simulink model "overcurrentest"  (R2019b)
settings: Solver=ode45  StartTime=0.0  StopTime=1.0  RelTol=1e-3  AbsTol=1e-6
undefined symbols (not defined in the file or in its folder): Time
libraries: elements x36
settings Model: ExtModeTrigMode=oneshot  ExtModeArmWhenConnect=off  Creator=PC  LastModifiedBy=taif205
settings SolverCC: AutoScaleAbsTol=off
settings DataIOCC: SaveFormat=Array  SignalLoggingSaveFormat=ModelDataLogs  ReturnWorkspaceOutputs=off
settings OptimizationCC: BlockReduction=off  BooleanDataType=off  LifeSpan=inf
settings DebuggingCC: SaveWithParameterizedLinksMsg=none  UnderspecifiedInitializationDetection=Classic  MergeDetectMultiDrivingBlocksExec=none  SignalResolutionControl=TryResolveAllWithWarning  MultiTaskDSMMsg=warning  MultiTaskCondExecSysMsg=none  SFUnexpectedBacktrackingDiag=warning  SFNoUnconditionalDefaultTransitionDiag=warning  SFExecutionAtInitializationDiag=none  ArithmeticOperatorsInVariantConditions=warning
settings HardwareCC: ProdBitPerPointer=32  ProdBitPerSizeT=32  ProdBitPerPtrDiffT=32  ProdLargestAtomicFloat=None  ProdIntDivRoundTo=Undefined  ProdEndianess=Unspecified  ProdWordSize=32  ProdHWDeviceType=32-bit Generic  TargetUnknown=on
settings ModelReferenceCC: PropagateSignalLabelsOutOfModel=off
settings SFSimCC: SimUseLocalCustomCode=off  CustomCodeUndefinedFunction=UseInterfaceOnly
settings RTWCC: RTWUseLocalCustomCode=off
settings CodeAppCC: StateflowObjectComments=on
settings GRTTargetCC: TargetLangStandard=C89/C90 (ANSI)  GeneratePreprocessorConditionals=Disable all  CombineOutputUpdateFcns=off  GRTInterface=on
settings ConfigComp: CovMetricSettings=dw  CovHtmlReporting=on  CovSaveCumulativeToWorkspaceVar=on  CovSaveSingleToWorkspaceVar=on  CovExternalEMLEnable=off

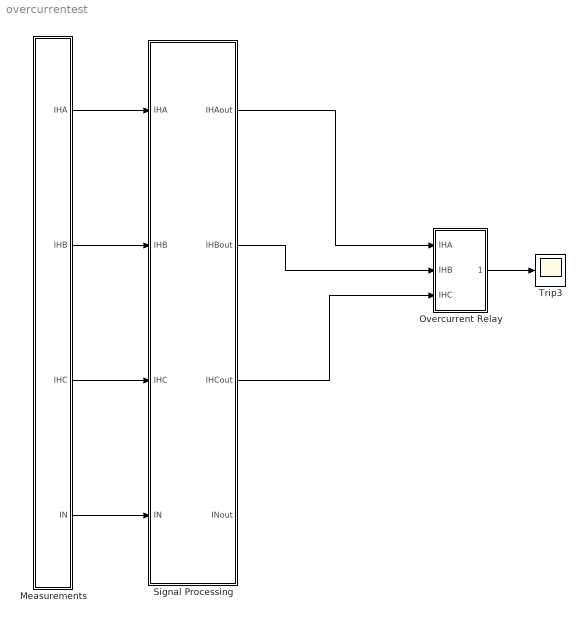
== system overcurrentest ==
  Measurements : Subsystem
  Overcurrent Relay : Subsystem  mask(Three-phase Inverse-time Overcurrent Relay){k=0.02, reset=0.9, pickupv=3}
      mask prompts: k "Time Parameter"; reset "Ratio of Reset to pick up"; pickupv "Pick-up Value"
      mask help: Three-phase inverse-time overcurrent relays for the back-up protection of the high voltage winding.
  Signal Processing : Subsystem  mask(Signal Processing){ctx=31.5, cth=1.38, vs=13.8e3, vp=315e3, vector=11}
      mask prompts: ctx "CT Ratio of Low Voltage Side"; cth "CT Ratio of High Voltage Side"; vs "Secondary Voltage"; vp "Primary Voltage"; vector "Transformer Connection Vector"
      mask help: Transform analog measurements to digital format, including filtering, sampling . . .
  Trip3 : Scope
  wires:
  Measurements/1(IHA) -> Signal Processing/1(IHA)
  Measurements/2(IHB) -> Signal Processing/2(IHB)
  Measurements/3(IHC) -> Signal Processing/3(IHC)
  Measurements/4(IN) -> Signal Processing/4(IN)
  Overcurrent Relay/1(Trip 3) -> Trip3/1
  Signal Processing/1(IHAout) -> Overcurrent Relay/1(IHA)
  Signal Processing/2(IHBout) -> Overcurrent Relay/2(IHB)
  Signal Processing/3(IHCout) -> Overcurrent Relay/3(IHC)

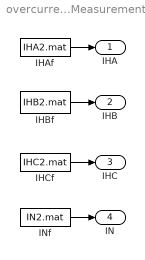
== system overcurrentest/Measurements ==
  IHAf : FromFile  FileName=IHA2.mat  SampleTime=0
  IHBf : FromFile  FileName=IHB2.mat  SampleTime=0
  IHCf : FromFile  FileName=IHC2.mat  SampleTime=0
  INf : FromFile  FileName=IN2.mat  SampleTime=0
  IHA : Outport
  IHB : Outport  Port=2
  IHC : Outport  Port=3
  IN : Outport  Port=4
  wires:
  IHAf/1 -> IHA/1
  IHBf/1 -> IHB/1
  IHCf/1 -> IHC/1
  INf/1 -> IN/1

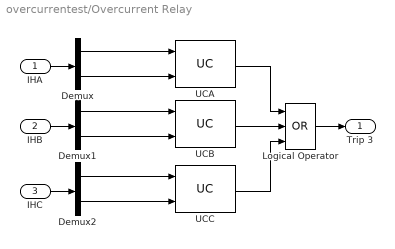
== system overcurrentest/Overcurrent Relay ==
  IHA : Inport
  IHB : Inport  Port=2
  IHC : Inport  Port=3
  Demux : Demux  Outputs=2
  Demux1 : Demux  Outputs=2
  Demux2 : Demux  Outputs=2
  Logical Operator : Logic  Operator=OR  Inputs=3
  UCA : elements/UC  type0=Signal-Time  sign=>  Ipickup=pickupv  k1=reset  type1=Very Inverse  type3=integration  k=k  fs=32*60
  UCB : elements/UC  type0=Signal-Time  sign=>  Ipickup=pickupv  k1=reset  type1=Very Inverse  type3=integration  k=k  fs=32*60
  UCC : elements/UC  type0=Signal-Time  sign=>  Ipickup=pickupv  k1=reset  type1=Very Inverse  type3=integration  k=k  fs=32*60
  Trip 3 : Outport
  wires:
  Demux2/1 -> UCC/1
  Demux1/1 -> UCB/1
  Demux/1 -> UCA/1
  UCA/1 -> Logical Operator/1
  UCB/1 -> Logical Operator/2
  UCC/1 -> Logical Operator/3
  Logical Operator/1 -> Trip 3/1
  IHA/1 -> Demux/1
  IHB/1 -> Demux1/1
  IHC/1 -> Demux2/1
  Demux/2 -> UCA/2
  Demux1/2 -> UCB/2
  Demux2/2 -> UCC/2

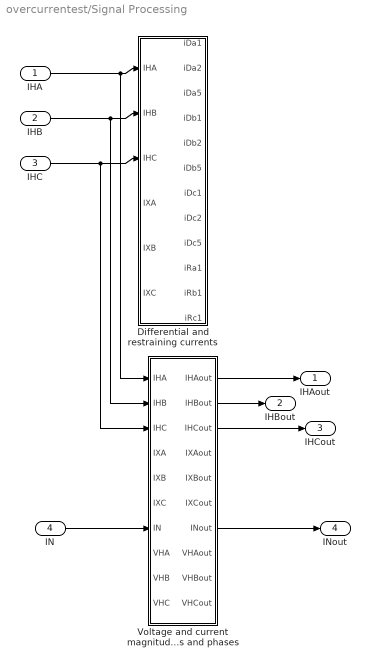
== system overcurrentest/Signal Processing ==
  IHA : Inport
  IHB : Inport  Port=2
  IHC : Inport  Port=3
  IN : Inport  Port=4
  Differential and restraining currents : Subsystem
  Voltage and current magnitudes and phases : Subsystem
  IHAout : Outport
  IHBout : Outport  Port=2
  IHCout : Outport  Port=3
  INout : Outport  Port=4
  wires:
  IHA/1 -> Differential and restraining currents/1(IHA), Voltage and current magnitudes and phases/1(IHA)
  IHB/1 -> Differential and restraining currents/2(IHB), Voltage and current magnitudes and phases/2(IHB)
  IHC/1 -> Differential and restraining currents/3(IHC), Voltage and current magnitudes and phases/3(IHC)
  Voltage and current magnitudes and phases/1(IHAout) -> IHAout/1
  Voltage and current magnitudes and phases/2(IHBout) -> IHBout/1
  Voltage and current magnitudes and phases/3(IHCout) -> IHCout/1
  Voltage and current magnitudes and phases/7(INout) -> INout/1
  IN/1 -> Voltage and current magnitudes and phases/7(IN)

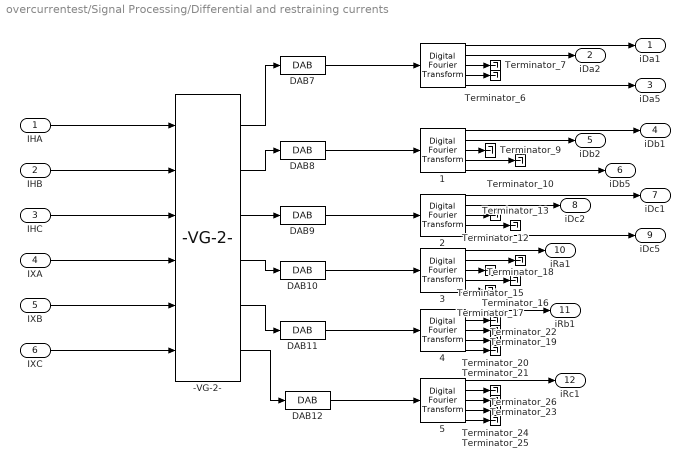
== system overcurrentest/Signal Processing/Differential and restraining currents ==
  IHA : Inport
  IHB : Inport  Port=2
  IHC : Inport  Port=3
  IXA : Inport  Port=4
  IXB : Inport  Port=5
  IXC : Inport  Port=6
   {,1..5} (6 alike) : elements/   fo=60  window_size=32  harmonic=[1 2 3 4 5]
  -VG-2- : elements/-VG-2-  trtype=wye - delta  vector=11  Vh=vp  Vx=vs  nCTH=cth  nCTX=ctx
  DAB{8..12} (5 alike) : elements/DAB  filter=off  approx=Bessel  order=2  numerator=[]  denominator=[]  freq=360  resdis=off  vertres=12  xmax=10  winsize=32  G=1.0  fs=60*32
  DAB7 : elements/DAB  filter=on  approx=Bessel  order=2  numerator=[]  denominator=[]  freq=360  resdis=off  vertres=12  xmax=10  winsize=32  G=1.0  fs=60*32
  Terminator_{6..7,9..10,12..13,15..26} (18 alike) : Terminator
  iDa1 : Outport
  iDa2 : Outport  Port=2
  iDa5 : Outport  Port=3
  iDb1 : Outport  Port=4
  iDb2 : Outport  Port=5
  iDb5 : Outport  Port=6
  iDc1 : Outport  Port=7
  iDc2 : Outport  Port=8
  iDc5 : Outport  Port=9
  iRa1 : Outport  Port=10
  iRb1 : Outport  Port=11
  iRc1 : Outport  Port=12
  wires:
  -VG-2-/1 -> DAB7/1
  -VG-2-/2 -> DAB8/1
  -VG-2-/3 -> DAB9/1
  -VG-2-/4 -> DAB10/1
  -VG-2-/5 -> DAB11/1
  -VG-2-/6 -> DAB12/1
  " 2"/3 -> Terminator_12/1
  " 2"/4 -> Terminator_13/1
  " 4"/5 -> Terminator_21/1
  DAB9/1 -> " 2"/1
  " 5"/2 -> Terminator_26/1
  " 5"/3 -> Terminator_23/1
  " 5"/4 -> Terminator_24/1
  " 5"/5 -> Terminator_25/1
  DAB12/1 -> " 5"/1
  " 4"/3 -> Terminator_19/1
  " 4"/2 -> Terminator_22/1
  DAB11/1 -> " 4"/1
  " 4"/4 -> Terminator_20/1
  " 3"/3 -> Terminator_15/1
  " 3"/4 -> Terminator_16/1
  " 3"/5 -> Terminator_17/1
  " 3"/2 -> Terminator_18/1
  DAB10/1 -> " 3"/1
  " 2"/1 -> iDc1/1
  " 2"/2 -> iDc2/1
  " 2"/5 -> iDc5/1
  " 3"/1 -> iRa1/1
  " 4"/1 -> iRb1/1
  " 5"/1 -> iRc1/1
  IXC/1 -> -VG-2-/6
  IXB/1 -> -VG-2-/5
  IXA/1 -> -VG-2-/4
  IHC/1 -> -VG-2-/3
  IHB/1 -> -VG-2-/2
  IHA/1 -> -VG-2-/1
  " "/4 -> Terminator_6/1
  " "/3 -> Terminator_7/1
  DAB7/1 -> " "/1
  " "/1 -> iDa1/1
  " "/2 -> iDa2/1
  " "/5 -> iDa5/1
  " 1"/3 -> Terminator_9/1
  " 1"/4 -> Terminator_10/1
  " 1"/1 -> iDb1/1
  " 1"/2 -> iDb2/1
  " 1"/5 -> iDb5/1
  DAB8/1 -> " 1"/1

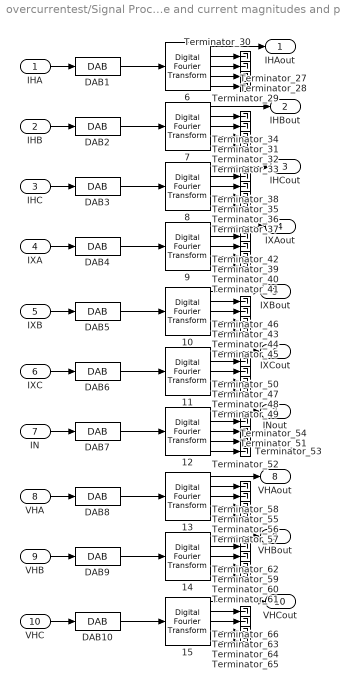
== system overcurrentest/Signal Processing/Voltage and current magnitudes and phases ==
  IHA : Inport
  IHB : Inport  Port=2
  IHC : Inport  Port=3
  IXA : Inport  Port=4
  IXB : Inport  Port=5
  IXC : Inport  Port=6
  IN : Inport  Port=7
  VHA : Inport  Port=8
  VHB : Inport  Port=9
  VHC : Inport  Port=10
   {6..15} (10 alike) : elements/   fo=60  window_size=32  harmonic=[1 2 3 4 5]
  DAB{1..10} (10 alike) : elements/DAB  filter=off  approx=Bessel  order=2  numerator=[]  denominator=[]  freq=360  resdis=off  vertres=12  xmax=10  winsize=32  G=1.0  fs=60*32
  Terminator_{27..66} (40 alike) : Terminator
  IHAout : Outport
  IHBout : Outport  Port=2
  IHCout : Outport  Port=3
  IXAout : Outport  Port=4
  IXBout : Outport  Port=5
  IXCout : Outport  Port=6
  INout : Outport  Port=7
  VHAout : Outport  Port=8
  VHBout : Outport  Port=9
  VHCout : Outport  Port=10
  wires:
  " 6"/2 -> Terminator_30/1
  " 6"/3 -> Terminator_27/1
  " 6"/4 -> Terminator_28/1
  " 6"/5 -> Terminator_29/1
  DAB1/1 -> " 6"/1
  IHA/1 -> DAB1/1
  " 7"/2 -> Terminator_34/1
  " 7"/3 -> Terminator_31/1
  " 7"/4 -> Terminator_32/1
  " 7"/5 -> Terminator_33/1
  DAB2/1 -> " 7"/1
  " 8"/2 -> Terminator_38/1
  " 8"/3 -> Terminator_35/1
  " 8"/4 -> Terminator_36/1
  " 8"/5 -> Terminator_37/1
  DAB3/1 -> " 8"/1
  " 9"/2 -> Terminator_42/1
  " 9"/3 -> Terminator_39/1
  " 9"/4 -> Terminator_40/1
  " 9"/5 -> Terminator_41/1
  DAB4/1 -> " 9"/1
  " 10"/2 -> Terminator_46/1
  " 10"/3 -> Terminator_43/1
  " 10"/4 -> Terminator_44/1
  " 10"/5 -> Terminator_45/1
  DAB5/1 -> " 10"/1
  " 11"/2 -> Terminator_50/1
  " 11"/3 -> Terminator_47/1
  " 11"/4 -> Terminator_48/1
  " 11"/5 -> Terminator_49/1
  DAB6/1 -> " 11"/1
  " 12"/2 -> Terminator_54/1
  " 12"/3 -> Terminator_51/1
  " 12"/4 -> Terminator_52/1
  " 12"/5 -> Terminator_53/1
  DAB7/1 -> " 12"/1
  " 13"/2 -> Terminator_58/1
  " 13"/3 -> Terminator_55/1
  " 13"/4 -> Terminator_56/1
  " 13"/5 -> Terminator_57/1
  DAB8/1 -> " 13"/1
  " 14"/2 -> Terminator_62/1
  " 14"/3 -> Terminator_59/1
  " 14"/4 -> Terminator_60/1
  " 14"/5 -> Terminator_61/1
  DAB9/1 -> " 14"/1
  " 15"/2 -> Terminator_66/1
  " 15"/3 -> Terminator_63/1
  " 15"/4 -> Terminator_64/1
  " 15"/5 -> Terminator_65/1
  DAB10/1 -> " 15"/1
  " 6"/1 -> IHAout/1
  " 7"/1 -> IHBout/1
  IHB/1 -> DAB2/1
  " 8"/1 -> IHCout/1
  IHC/1 -> DAB3/1
  " 9"/1 -> IXAout/1
  IXA/1 -> DAB4/1
  " 10"/1 -> IXBout/1
  IXB/1 -> DAB5/1
  " 11"/1 -> IXCout/1
  IXC/1 -> DAB6/1
  " 12"/1 -> INout/1
  IN/1 -> DAB7/1
  " 13"/1 -> VHAout/1
  VHA/1 -> DAB8/1
  " 14"/1 -> VHBout/1
  VHB/1 -> DAB9/1
  " 15"/1 -> VHCout/1
  VHC/1 -> DAB10/1
